simulink model "oving3_a_m_skallfil"  (R2023a)
settings: Solver=VariableStepAuto  StartTime=0.0  StopTime=3  FixedStep=.4  RelTol=1e-3
settings Model: Creator=tormod  LastModifiedBy=tormod
settings DebuggingCC: UnconnectedInputMsg=warning  UnconnectedOutputMsg=warning  UnconnectedLineMsg=warning
settings ModelReferenceCC: EnableRefExpFcnMdlSchedulingChecks=on
settings RTWCC: DLArmComputeVersion=19.05

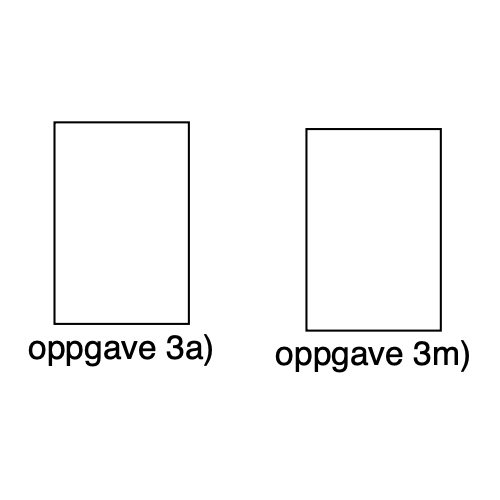
[thumbnail: Simulink's stored preview of the top-level diagram]
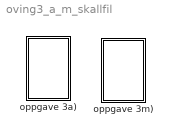
== system oving3_a_m_skallfil ==
  oppgave 3a) : Subsystem
  oppgave 3m) : Subsystem

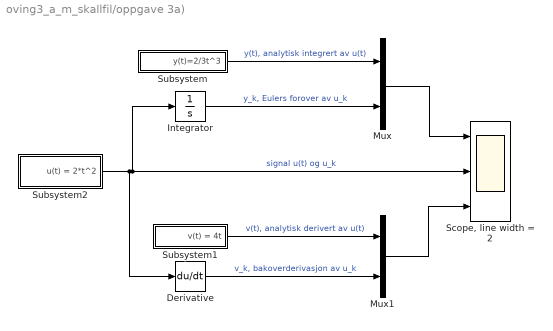
== system oving3_a_m_skallfil/oppgave 3a) ==
  Derivative : Derivative
  Integrator : Integrator
      settings: AttributesFormatString=IC = %<InitialCondition>
  Mux : Mux  Inputs=2
  Mux1 : Mux  Inputs=2
  "Scope, line width = 2" : Scope  NumInputPorts=3
  Subsystem : Subsystem
  Subsystem1 : Subsystem
  Subsystem2 : Subsystem
  wires:
  Integrator/1 -> Mux/2  "y_k, Eulers forover av u_k"
  Derivative/1 -> Mux1/2  "v_k, bakoverderivasjon av u_k"
  Mux/1 -> "Scope, line width = 2"/1
  Mux1/1 -> "Scope, line width = 2"/3
  Subsystem/1(y(t)=2/3t^3) -> Mux/1  "y(t), analytisk integrert av u(t)"
  Subsystem1/1(v(t) = 4t) -> Mux1/1  "v(t), analytisk derivert av u(t)"
  Subsystem2/1(u(t) = 2*t^2) -> Derivative/1, "Scope, line width = 2"/2, Integrator/1  "signal u(t) og u_k"

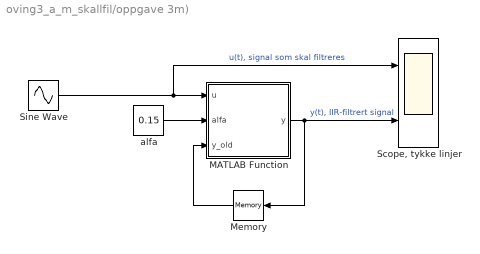
== system oving3_a_m_skallfil/oppgave 3m) ==
  MATLAB Function : MATLAB Function  TreatAsAtomicUnit=on
  Memory : Memory
      settings: AttributesFormatString=IC = %<InitialCondition>
  "Scope, tykke linjer" : Scope  NumInputPorts=2
  Sine Wave : Sin  Amplitude=0.1  Bias=0.2  Frequency=0.628  SampleTime=0
      settings: AttributesFormatString=u(t) = %<Amplitude> sin(%<Frequency>t + %<Phase>) + %<Bias>
  alfa : Constant  Value=0.15
  wires:
  Sine Wave/1 -> "Scope, tykke linjer"/1, MATLAB Function/1(u)  "u(t), signal som skal filtreres"
  Memory/1 -> MATLAB Function/3(y_old)
  alfa/1 -> MATLAB Function/2(alfa)
  MATLAB Function/1(y) -> "Scope, tykke linjer"/2, Memory/1  "y(t), IIR-filtrert signal"

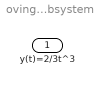
== system oving3_a_m_skallfil/oppgave 3a)/Subsystem ==
  y(t)=2/3t^3 : Outport
  wires:
  ? -> y(t)=2/3t^3/1  "y(t), integrert av u(t)"

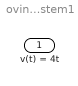
== system oving3_a_m_skallfil/oppgave 3a)/Subsystem1 ==
  v(t) = 4t : Outport
  wires:
  ? -> v(t) = 4t/1  "v(t), derivert av u(t)"

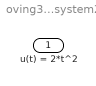
== system oving3_a_m_skallfil/oppgave 3a)/Subsystem2 ==
  u(t) = 2*t^2 : Outport
  wires:
  ? -> u(t) = 2*t^2/1  "signal u(t)"

== matlab function oving3_a_m_skallfil/oppgave 3m)/MATLAB Function ==
  data: u input; alfa input; y output; y_old input
function y = fcn(u,alfa,y_old)

y = 1; % erstatt denne med kode
